simulink model "uz_sine_generator_16bit"  (R2023a)
settings: Solver=FixedStepDiscrete  StartTime=0.0  StopTime=50000/100e6  RelTol=1e-3
libraries: hdlsllib x17, embmathops x8, simulink x1
settings Model: DataTypeOverride=Off  Creator=ts  LastModifiedBy=ts
settings SolverCC: AlgebraicLoopSolver=TrustRegion
settings DataIOCC: LimitDataPoints=on  SaveOutput=off  SaveTime=off
settings OptimizationCC: BlockReduction=off  ConditionallyExecuteInputs=off  DefaultParameterBehavior=Inlined  LifeSpan=inf
settings DebuggingCC: AlgebraicLoopMsg=error  SingleTaskRateTransMsg=error  UnconnectedInputMsg=warning  UnconnectedOutputMsg=warning  UnconnectedLineMsg=warning  AllowSymbolicDim=off  StrictBusMsg=ErrorOnBusTreatedAsVector  SFUnexpectedBacktrackingDiag=warning  SFNoUnconditionalDefaultTransitionDiag=warning  SFExecutionAtInitializationDiag=none  ArithmeticOperatorsInVariantConditions=warning
settings HardwareCC: ProdBitPerPointer=32  ProdBitPerSizeT=32  ProdBitPerPtrDiffT=32  ProdLargestAtomicFloat=None  ProdIntDivRoundTo=Undefined  ProdEndianess=Unspecified  ProdWordSize=32  ProdHWDeviceType=ASIC/FPGA->ASIC/FPGA  ProdEqTarget=off
settings ModelReferenceCC: EnableRefExpFcnMdlSchedulingChecks=on
settings SFSimCC: SimUseLocalCustomCode=off  CustomCodeUndefinedFunction=UseInterfaceOnly
settings RTWCC: RTWUseLocalCustomCode=off
settings CodeAppCC: StateflowObjectComments=on
settings GRTTargetCC: TargetLangStandard=C89/C90 (ANSI)
settings ConfigComp: CovScope=ReferencedModels  CovMetricSettings=dw  CovSaveCumulativeToWorkspaceVar=on  CovSaveSingleToWorkspaceVar=on  CovExternalEMLEnable=off  CovSFcnEnable=off

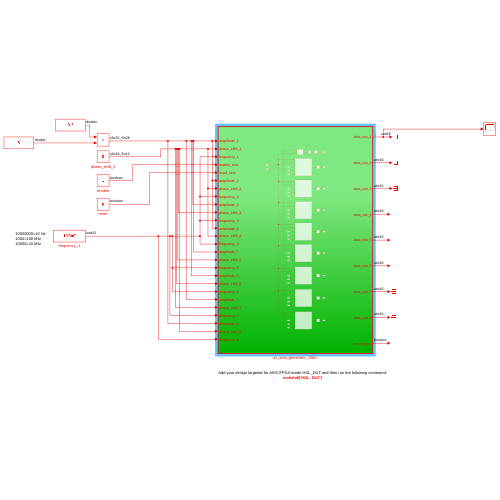
[thumbnail: Simulink's stored preview of the top-level diagram]
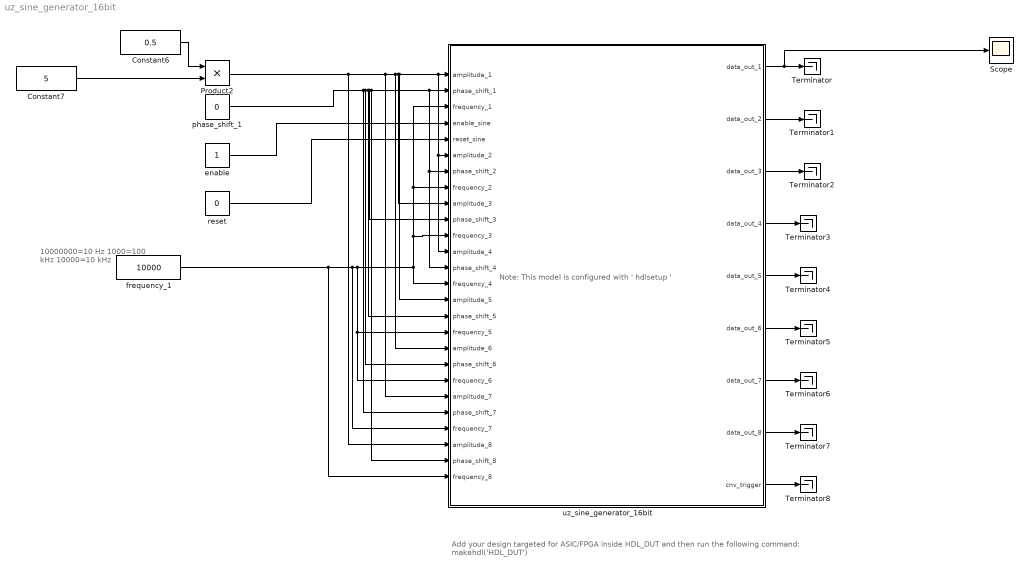
== system uz_sine_generator_16bit ==
  note: Note: This model is configured with ' hdlsetup '
  note: Add your design targeted for ASIC/FPGA inside HDL_DUT and then run the following command:
      | makehdl('HDL_DUT')
  note: 10000000=10 Hz
      | 1000=100 kHz
      | 10000=10 kHz
  Constant6 : Constant  Value=0.5  SampleTime=-1
  Constant7 : Constant  Value=5  SampleTime=-1
  Product2 : Product  OutDataTypeStr=fixdt(1,32,28)
  Scope : Scope
  Terminator{,1..8} (9 alike) : Terminator
  enable : Constant  OutDataTypeStr=boolean  SampleTime=-1
  frequency_1 : Constant  Value=10000  OutDataTypeStr=uint32  SampleTime=1/100e6
  phase_shift_1 : Constant  Value=0  OutDataTypeStr=fixdt(1,16,12)  SampleTime=-1
  reset : Constant  Value=0  OutDataTypeStr=boolean  SampleTime=-1
  "uz_sine_generator_16bit " : Subsystem  TreatAsAtomicUnit=on
  wires:
  Constant6/1 -> Product2/1
  Constant7/1 -> Product2/2
  Product2/1 -> "uz_sine_generator_16bit "/24(amplitude_8), "uz_sine_generator_16bit "/21(amplitude_7), "uz_sine_generator_16bit "/18(amplitude_6), "uz_sine_generator_16bit "/9(amplitude_3), "uz_sine_generator_16bit "/15(amplitude_5), "uz_sine_generator_16bit "/12(amplitude_4), "uz_sine_generator_16bit "/6(amplitude_2), "uz_sine_generator_16bit "/1(amplitude_1)
  phase_shift_1/1 -> "uz_sine_generator_16bit "/25(phase_shift_8), "uz_sine_generator_16bit "/13(phase_shift_4), "uz_sine_generator_16bit "/7(phase_shift_2), "uz_sine_generator_16bit "/2(phase_shift_1), "uz_sine_generator_16bit "/10(phase_shift_3), "uz_sine_generator_16bit "/16(phase_shift_5), "uz_sine_generator_16bit "/19(phase_shift_6), "uz_sine_generator_16bit "/22(phase_shift_7)
  "uz_sine_generator_16bit "/1(data_out_1) -> Scope/1, Terminator/1
  "uz_sine_generator_16bit "/2(data_out_2) -> Terminator1/1
  "uz_sine_generator_16bit "/3(data_out_3) -> Terminator2/1
  "uz_sine_generator_16bit "/4(data_out_4) -> Terminator3/1
  "uz_sine_generator_16bit "/5(data_out_5) -> Terminator4/1
  "uz_sine_generator_16bit "/6(data_out_6) -> Terminator5/1
  "uz_sine_generator_16bit "/7(data_out_7) -> Terminator6/1
  "uz_sine_generator_16bit "/8(data_out_8) -> Terminator7/1
  "uz_sine_generator_16bit "/9(cnv_trigger) -> Terminator8/1
  enable/1 -> "uz_sine_generator_16bit "/4(enable_sine)
  reset/1 -> "uz_sine_generator_16bit "/5(reset_sine)
  frequency_1/1 -> "uz_sine_generator_16bit "/26(frequency_8), "uz_sine_generator_16bit "/23(frequency_7), "uz_sine_generator_16bit "/20(frequency_6), "uz_sine_generator_16bit "/17(frequency_5), "uz_sine_generator_16bit "/14(frequency_4), "uz_sine_generator_16bit "/11(frequency_3), "uz_sine_generator_16bit "/3(frequency_1), "uz_sine_generator_16bit "/8(frequency_2)

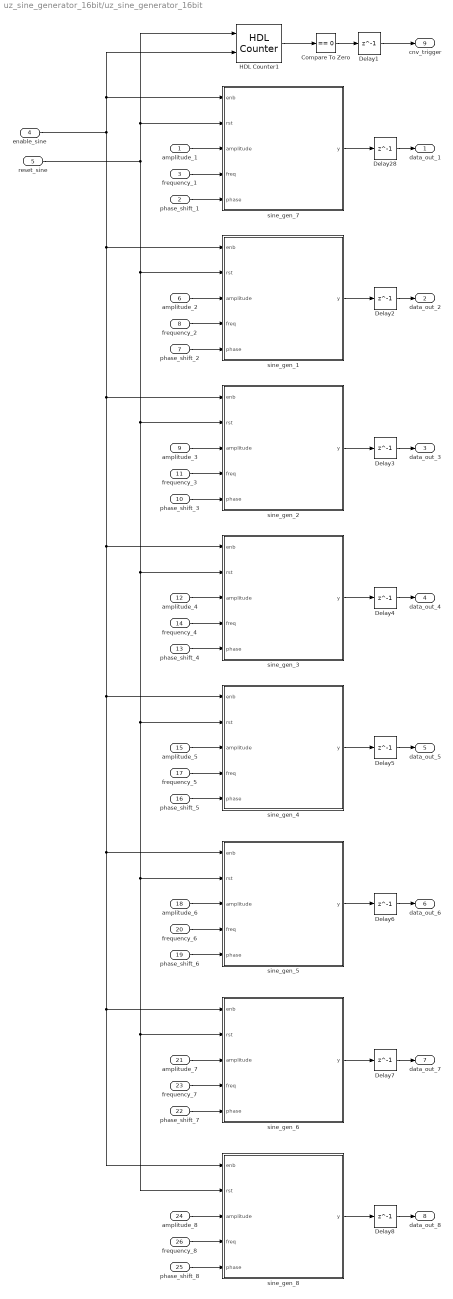
== system uz_sine_generator_16bit/uz_sine_generator_16bit  ==
  amplitude_1 : Inport
  phase_shift_1 : Inport  Port=2
  frequency_1 : Inport  Port=3
  enable_sine : Inport  Port=4
  reset_sine : Inport  Port=5
  amplitude_2 : Inport  Port=6
  phase_shift_2 : Inport  Port=7
  frequency_2 : Inport  Port=8
  amplitude_3 : Inport  Port=9
  phase_shift_3 : Inport  Port=10
  frequency_3 : Inport  Port=11
  amplitude_4 : Inport  Port=12
  phase_shift_4 : Inport  Port=13
  frequency_4 : Inport  Port=14
  amplitude_5 : Inport  Port=15
  phase_shift_5 : Inport  Port=16
  frequency_5 : Inport  Port=17
  amplitude_6 : Inport  Port=18
  phase_shift_6 : Inport  Port=19
  frequency_6 : Inport  Port=20
  amplitude_7 : Inport  Port=21
  phase_shift_7 : Inport  Port=22
  frequency_7 : Inport  Port=23
  amplitude_8 : Inport  Port=24
  phase_shift_8 : Inport  Port=25
  frequency_8 : Inport  Port=26
  Compare To Zero : simulink/Logic and Bit Operations/Compare To Zero  relop===  OutDataTypeStr=boolean
  Delay{1..8,28} (9 alike) : Delay  DelayLength=1
  HDL Counter1 : hdlsllib/Sources/HDL Counter  CountType=Free running  CountInit=0  CountStep=100  CountMax=25  CountFromType=Initial value  CountFrom=0  CountResetPort=on  CountLoadPort=off  CountEnbPort=on  CountDirPort=off  CountHitOutputPort=off  CountDataType=Unsigned  CountWordLen=8  CountFracLen=0  CountSampTime=1
  sine_gen_1 : Subsystem
  sine_gen_2 : Subsystem
  sine_gen_3 : Subsystem
  sine_gen_4 : Subsystem
  sine_gen_5 : Subsystem
  sine_gen_6 : Subsystem
  sine_gen_7 : Subsystem
  sine_gen_8 : Subsystem
  data_out_1 : Outport  VectorParamsAs1DForOutWhenUnconnected=off
  data_out_2 : Outport  Port=2  VectorParamsAs1DForOutWhenUnconnected=off
  data_out_3 : Outport  Port=3  VectorParamsAs1DForOutWhenUnconnected=off
  data_out_4 : Outport  Port=4  VectorParamsAs1DForOutWhenUnconnected=off
  data_out_5 : Outport  Port=5  VectorParamsAs1DForOutWhenUnconnected=off
  data_out_6 : Outport  Port=6  VectorParamsAs1DForOutWhenUnconnected=off
  data_out_7 : Outport  Port=7  VectorParamsAs1DForOutWhenUnconnected=off
  data_out_8 : Outport  Port=8  VectorParamsAs1DForOutWhenUnconnected=off
  cnv_trigger : Outport  Port=9  VectorParamsAs1DForOutWhenUnconnected=off
  wires:
  Delay28/1 -> data_out_1/1
  HDL Counter1/1 -> Compare To Zero/1
  Compare To Zero/1 -> Delay1/1
  sine_gen_7/1(y) -> Delay28/1
  amplitude_1/1 -> sine_gen_7/3(amplitude)
  Delay1/1 -> cnv_trigger/1
  amplitude_2/1 -> sine_gen_1/3(amplitude)
  sine_gen_1/1(y) -> Delay2/1
  Delay2/1 -> data_out_2/1
  amplitude_3/1 -> sine_gen_2/3(amplitude)
  sine_gen_2/1(y) -> Delay3/1
  Delay3/1 -> data_out_3/1
  amplitude_4/1 -> sine_gen_3/3(amplitude)
  sine_gen_3/1(y) -> Delay4/1
  Delay4/1 -> data_out_4/1
  amplitude_5/1 -> sine_gen_4/3(amplitude)
  sine_gen_4/1(y) -> Delay5/1
  Delay5/1 -> data_out_5/1
  amplitude_6/1 -> sine_gen_5/3(amplitude)
  sine_gen_5/1(y) -> Delay6/1
  Delay6/1 -> data_out_6/1
  amplitude_7/1 -> sine_gen_6/3(amplitude)
  sine_gen_6/1(y) -> Delay7/1
  Delay7/1 -> data_out_7/1
  amplitude_8/1 -> sine_gen_8/3(amplitude)
  sine_gen_8/1(y) -> Delay8/1
  enable_sine/1 -> sine_gen_7/1(enb), HDL Counter1/2, sine_gen_1/1(enb), sine_gen_2/1(enb), sine_gen_3/1(enb), sine_gen_4/1(enb), sine_gen_5/1(enb), sine_gen_8/1(enb), sine_gen_6/1(enb)
  reset_sine/1 -> sine_gen_1/2(rst), sine_gen_2/2(rst), sine_gen_3/2(rst), sine_gen_4/2(rst), sine_gen_5/2(rst), sine_gen_8/2(rst), sine_gen_6/2(rst), sine_gen_7/2(rst), HDL Counter1/1
  Delay8/1 -> data_out_8/1
  frequency_1/1 -> sine_gen_7/4(freq)
  phase_shift_1/1 -> sine_gen_7/5(phase)
  frequency_2/1 -> sine_gen_1/4(freq)
  phase_shift_2/1 -> sine_gen_1/5(phase)
  frequency_3/1 -> sine_gen_2/4(freq)
  phase_shift_3/1 -> sine_gen_2/5(phase)
  frequency_4/1 -> sine_gen_3/4(freq)
  phase_shift_4/1 -> sine_gen_3/5(phase)
  frequency_5/1 -> sine_gen_4/4(freq)
  phase_shift_5/1 -> sine_gen_4/5(phase)
  frequency_6/1 -> sine_gen_5/4(freq)
  phase_shift_6/1 -> sine_gen_5/5(phase)
  frequency_7/1 -> sine_gen_6/4(freq)
  phase_shift_7/1 -> sine_gen_6/5(phase)
  frequency_8/1 -> sine_gen_8/4(freq)
  phase_shift_8/1 -> sine_gen_8/5(phase)

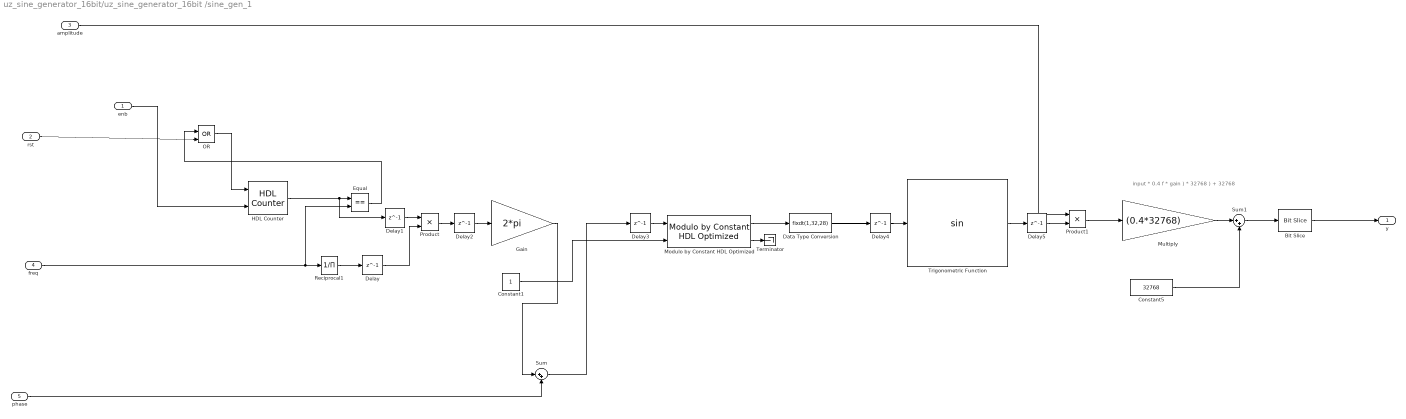
== system uz_sine_generator_16bit/uz_sine_generator_16bit /sine_gen_1 ==
  note: input * 0.4 f * gain ) * 32768 ) + 32768
  enb : Inport
  rst : Inport  Port=2
  amplitude : Inport  Port=3
  freq : Inport  Port=4
  phase : Inport  Port=5
  Bit Slice : hdlsllib/Logic and Bit Operations/Bit Slice  lidx=15  ridx=0
  Constant1 : Constant  OutDataTypeStr=boolean  SampleTime=-1
  Constant5 : Constant  Value=32768  OutDataTypeStr=int32  SampleTime=-1
  Data Type Conversion : DataTypeConversion  OutDataTypeStr=fixdt(1,32,28)  SaturateOnIntegerOverflow=off  RndMeth=Floor
  Delay{,1..5} (6 alike) : Delay  DelayLength=1
  Equal : RelationalOperator  Operator===  OutDataTypeStr=boolean  RndMeth=Simplest  InputSameDT=off
  Gain : Gain  Gain=2*pi  OutDataTypeStr=fixdt(1,32,28)
  HDL Counter : hdlsllib/Sources/HDL Counter  CountType=Free running  CountInit=0  CountStep=1  CountMax=25  CountFromType=Initial value  CountFrom=0  CountResetPort=on  CountLoadPort=off  CountEnbPort=on  CountDirPort=off  CountHitOutputPort=off  CountDataType=Unsigned  CountWordLen=32  CountFracLen=0  CountSampTime=1
  Modulo by Constant HDL Optimized : embmathops/Modulo by Constant HDL Optimized  Denominator=2*pi  SimulateUsing=Code generation
      settings: LibrarySourceBlock=|
      | embeddedMatrixLib/Math Operations/Modulo by Constant
      | HDL Optimized
  Multiply : Gain  Gain=(0.4*32768)  OutDataTypeStr=int32
  OR : Logic  Operator=OR  IconShape=distinctive  AllPortsSameDT=off  OutDataTypeStr=boolean
  Product : Product  OutDataTypeStr=fixdt(0,32,29)
  Product1 : Product  OutDataTypeStr=Inherit: Same as first input
  Reciprocal1 : Product  Inputs=/  RndMeth=Zero  SaturateOnIntegerOverflow=on
  Sum : Sum  Inputs=|++
  Sum1 : Sum  Inputs=|++  OutDataTypeStr=int32
  Terminator : Terminator
  Trigonometric Function : Trigonometry  ApproximationMethod=CORDIC
  y : Outport
  wires:
  Constant1/1 -> Modulo by Constant HDL Optimized/2
  Product1/1 -> Multiply/1
  Constant5/1 -> Sum1/2
  Gain/1 -> Sum/1
  Sum/1 -> Delay3/1
  Modulo by Constant HDL Optimized/1 -> Data Type Conversion/1
  freq/1 -> Reciprocal1/1, Equal/2
  Reciprocal1/1 -> Delay/1
  amplitude/1 -> Product1/1
  Sum1/1 -> Bit Slice/1
  phase/1 -> Sum/2
  Product/1 -> Delay2/1
  Equal/1 -> OR/1
  Trigonometric Function/1 -> Delay5/1
  enb/1 -> HDL Counter/2
  Multiply/1 -> Sum1/1
  Bit Slice/1 -> y/1
  Modulo by Constant HDL Optimized/2 -> Terminator/1
  OR/1 -> HDL Counter/1
  rst/1 -> OR/2
  HDL Counter/1 -> Delay1/1, Equal/1
  Data Type Conversion/1 -> Delay4/1
  Delay/1 -> Product/2
  Delay1/1 -> Product/1
  Delay2/1 -> Gain/1
  Delay3/1 -> Modulo by Constant HDL Optimized/1
  Delay4/1 -> Trigonometric Function/1
  Delay5/1 -> Product1/2

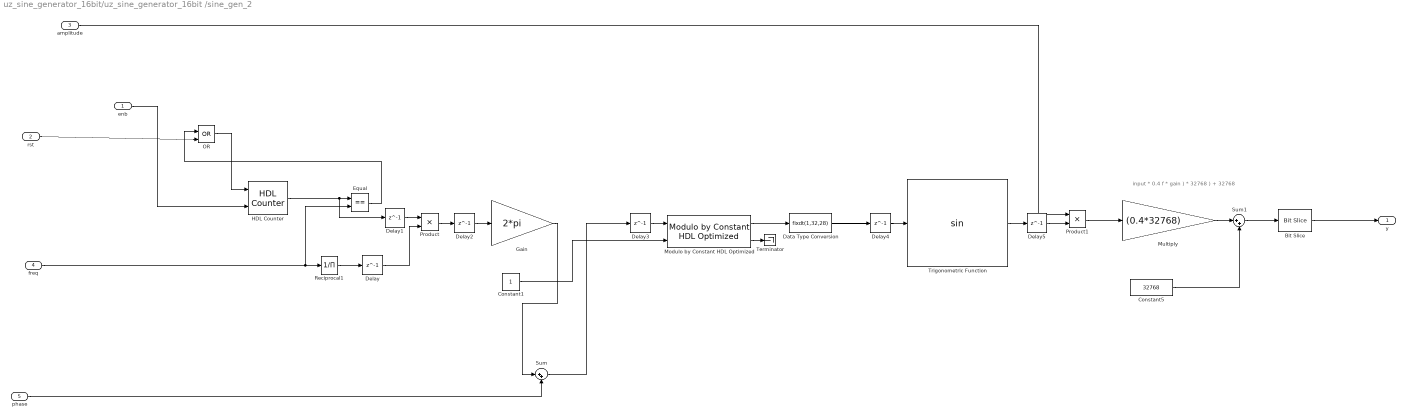
== system uz_sine_generator_16bit/uz_sine_generator_16bit /sine_gen_2 ==
  note: input * 0.4 f * gain ) * 32768 ) + 32768
  enb : Inport
  rst : Inport  Port=2
  amplitude : Inport  Port=3
  freq : Inport  Port=4
  phase : Inport  Port=5
  Bit Slice : hdlsllib/Logic and Bit Operations/Bit Slice  lidx=15  ridx=0
  Constant1 : Constant  OutDataTypeStr=boolean  SampleTime=-1
  Constant5 : Constant  Value=32768  OutDataTypeStr=int32  SampleTime=-1
  Data Type Conversion : DataTypeConversion  OutDataTypeStr=fixdt(1,32,28)  SaturateOnIntegerOverflow=off  RndMeth=Floor
  Delay{,1..5} (6 alike) : Delay  DelayLength=1
  Equal : RelationalOperator  Operator===  OutDataTypeStr=boolean  RndMeth=Simplest  InputSameDT=off
  Gain : Gain  Gain=2*pi  OutDataTypeStr=fixdt(1,32,28)
  HDL Counter : hdlsllib/Sources/HDL Counter  CountType=Free running  CountInit=0  CountStep=1  CountMax=25  CountFromType=Initial value  CountFrom=0  CountResetPort=on  CountLoadPort=off  CountEnbPort=on  CountDirPort=off  CountHitOutputPort=off  CountDataType=Unsigned  CountWordLen=32  CountFracLen=0  CountSampTime=1
  Modulo by Constant HDL Optimized : embmathops/Modulo by Constant HDL Optimized  Denominator=2*pi  SimulateUsing=Code generation
      settings: LibrarySourceBlock=|
      | embeddedMatrixLib/Math Operations/Modulo by Constant
      | HDL Optimized
  Multiply : Gain  Gain=(0.4*32768)  OutDataTypeStr=int32
  OR : Logic  Operator=OR  IconShape=distinctive  AllPortsSameDT=off  OutDataTypeStr=boolean
  Product : Product  OutDataTypeStr=fixdt(0,32,29)
  Product1 : Product  OutDataTypeStr=Inherit: Same as first input
  Reciprocal1 : Product  Inputs=/  RndMeth=Zero  SaturateOnIntegerOverflow=on
  Sum : Sum  Inputs=|++
  Sum1 : Sum  Inputs=|++  OutDataTypeStr=int32
  Terminator : Terminator
  Trigonometric Function : Trigonometry  ApproximationMethod=CORDIC
  y : Outport
  wires:
  Constant1/1 -> Modulo by Constant HDL Optimized/2
  Product1/1 -> Multiply/1
  Constant5/1 -> Sum1/2
  Gain/1 -> Sum/1
  Sum/1 -> Delay3/1
  Modulo by Constant HDL Optimized/1 -> Data Type Conversion/1
  freq/1 -> Reciprocal1/1, Equal/2
  Reciprocal1/1 -> Delay/1
  amplitude/1 -> Product1/1
  Sum1/1 -> Bit Slice/1
  phase/1 -> Sum/2
  Product/1 -> Delay2/1
  Equal/1 -> OR/1
  Trigonometric Function/1 -> Delay5/1
  enb/1 -> HDL Counter/2
  Multiply/1 -> Sum1/1
  Bit Slice/1 -> y/1
  Modulo by Constant HDL Optimized/2 -> Terminator/1
  OR/1 -> HDL Counter/1
  rst/1 -> OR/2
  HDL Counter/1 -> Delay1/1, Equal/1
  Data Type Conversion/1 -> Delay4/1
  Delay/1 -> Product/2
  Delay1/1 -> Product/1
  Delay2/1 -> Gain/1
  Delay3/1 -> Modulo by Constant HDL Optimized/1
  Delay4/1 -> Trigonometric Function/1
  Delay5/1 -> Product1/2

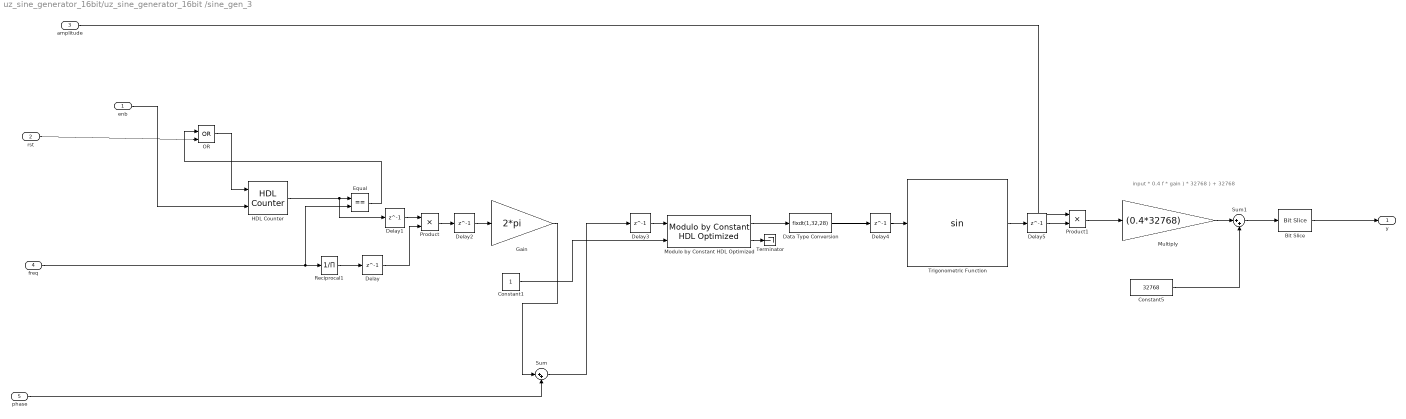
== system uz_sine_generator_16bit/uz_sine_generator_16bit /sine_gen_3 ==
  note: input * 0.4 f * gain ) * 32768 ) + 32768
  enb : Inport
  rst : Inport  Port=2
  amplitude : Inport  Port=3
  freq : Inport  Port=4
  phase : Inport  Port=5
  Bit Slice : hdlsllib/Logic and Bit Operations/Bit Slice  lidx=15  ridx=0
  Constant1 : Constant  OutDataTypeStr=boolean  SampleTime=-1
  Constant5 : Constant  Value=32768  OutDataTypeStr=int32  SampleTime=-1
  Data Type Conversion : DataTypeConversion  OutDataTypeStr=fixdt(1,32,28)  SaturateOnIntegerOverflow=off  RndMeth=Floor
  Delay{,1..5} (6 alike) : Delay  DelayLength=1
  Equal : RelationalOperator  Operator===  OutDataTypeStr=boolean  RndMeth=Simplest  InputSameDT=off
  Gain : Gain  Gain=2*pi  OutDataTypeStr=fixdt(1,32,28)
  HDL Counter : hdlsllib/Sources/HDL Counter  CountType=Free running  CountInit=0  CountStep=1  CountMax=25  CountFromType=Initial value  CountFrom=0  CountResetPort=on  CountLoadPort=off  CountEnbPort=on  CountDirPort=off  CountHitOutputPort=off  CountDataType=Unsigned  CountWordLen=32  CountFracLen=0  CountSampTime=1
  Modulo by Constant HDL Optimized : embmathops/Modulo by Constant HDL Optimized  Denominator=2*pi  SimulateUsing=Code generation
      settings: LibrarySourceBlock=|
      | embeddedMatrixLib/Math Operations/Modulo by Constant
      | HDL Optimized
  Multiply : Gain  Gain=(0.4*32768)  OutDataTypeStr=int32
  OR : Logic  Operator=OR  IconShape=distinctive  AllPortsSameDT=off  OutDataTypeStr=boolean
  Product : Product  OutDataTypeStr=fixdt(0,32,29)
  Product1 : Product  OutDataTypeStr=Inherit: Same as first input
  Reciprocal1 : Product  Inputs=/  RndMeth=Zero  SaturateOnIntegerOverflow=on
  Sum : Sum  Inputs=|++
  Sum1 : Sum  Inputs=|++  OutDataTypeStr=int32
  Terminator : Terminator
  Trigonometric Function : Trigonometry  ApproximationMethod=CORDIC
  y : Outport
  wires:
  Constant1/1 -> Modulo by Constant HDL Optimized/2
  Product1/1 -> Multiply/1
  Constant5/1 -> Sum1/2
  Gain/1 -> Sum/1
  Sum/1 -> Delay3/1
  Modulo by Constant HDL Optimized/1 -> Data Type Conversion/1
  freq/1 -> Reciprocal1/1, Equal/2
  Reciprocal1/1 -> Delay/1
  amplitude/1 -> Product1/1
  Sum1/1 -> Bit Slice/1
  phase/1 -> Sum/2
  Product/1 -> Delay2/1
  Equal/1 -> OR/1
  Trigonometric Function/1 -> Delay5/1
  enb/1 -> HDL Counter/2
  Multiply/1 -> Sum1/1
  Bit Slice/1 -> y/1
  Modulo by Constant HDL Optimized/2 -> Terminator/1
  OR/1 -> HDL Counter/1
  rst/1 -> OR/2
  HDL Counter/1 -> Delay1/1, Equal/1
  Data Type Conversion/1 -> Delay4/1
  Delay/1 -> Product/2
  Delay1/1 -> Product/1
  Delay2/1 -> Gain/1
  Delay3/1 -> Modulo by Constant HDL Optimized/1
  Delay4/1 -> Trigonometric Function/1
  Delay5/1 -> Product1/2

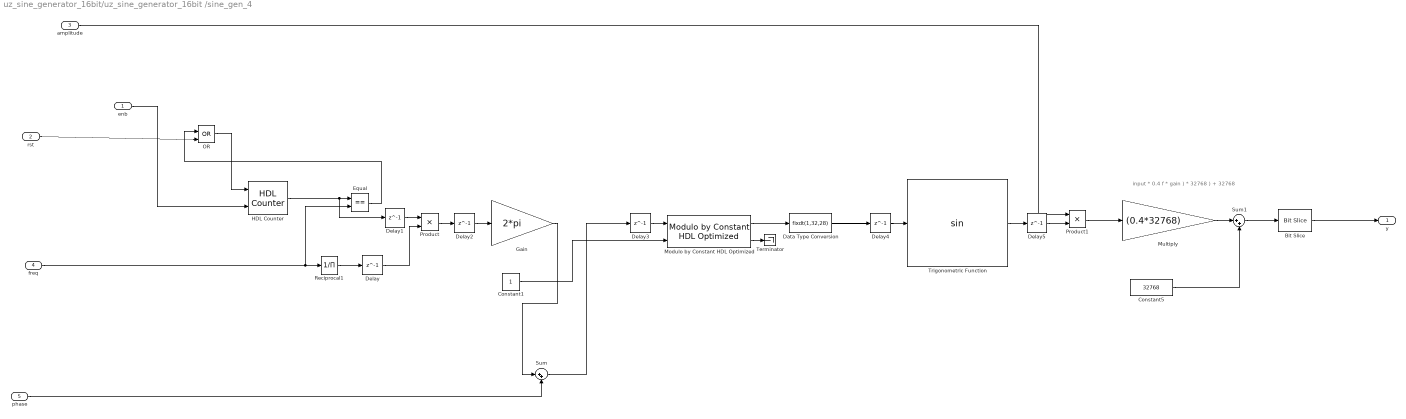
== system uz_sine_generator_16bit/uz_sine_generator_16bit /sine_gen_4 ==
  note: input * 0.4 f * gain ) * 32768 ) + 32768
  enb : Inport
  rst : Inport  Port=2
  amplitude : Inport  Port=3
  freq : Inport  Port=4
  phase : Inport  Port=5
  Bit Slice : hdlsllib/Logic and Bit Operations/Bit Slice  lidx=15  ridx=0
  Constant1 : Constant  OutDataTypeStr=boolean  SampleTime=-1
  Constant5 : Constant  Value=32768  OutDataTypeStr=int32  SampleTime=-1
  Data Type Conversion : DataTypeConversion  OutDataTypeStr=fixdt(1,32,28)  SaturateOnIntegerOverflow=off  RndMeth=Floor
  Delay{,1..5} (6 alike) : Delay  DelayLength=1
  Equal : RelationalOperator  Operator===  OutDataTypeStr=boolean  RndMeth=Simplest  InputSameDT=off
  Gain : Gain  Gain=2*pi  OutDataTypeStr=fixdt(1,32,28)
  HDL Counter : hdlsllib/Sources/HDL Counter  CountType=Free running  CountInit=0  CountStep=1  CountMax=25  CountFromType=Initial value  CountFrom=0  CountResetPort=on  CountLoadPort=off  CountEnbPort=on  CountDirPort=off  CountHitOutputPort=off  CountDataType=Unsigned  CountWordLen=32  CountFracLen=0  CountSampTime=1
  Modulo by Constant HDL Optimized : embmathops/Modulo by Constant HDL Optimized  Denominator=2*pi  SimulateUsing=Code generation
      settings: LibrarySourceBlock=|
      | embeddedMatrixLib/Math Operations/Modulo by Constant
      | HDL Optimized
  Multiply : Gain  Gain=(0.4*32768)  OutDataTypeStr=int32
  OR : Logic  Operator=OR  IconShape=distinctive  AllPortsSameDT=off  OutDataTypeStr=boolean
  Product : Product  OutDataTypeStr=fixdt(0,32,29)
  Product1 : Product  OutDataTypeStr=Inherit: Same as first input
  Reciprocal1 : Product  Inputs=/  RndMeth=Zero  SaturateOnIntegerOverflow=on
  Sum : Sum  Inputs=|++
  Sum1 : Sum  Inputs=|++  OutDataTypeStr=int32
  Terminator : Terminator
  Trigonometric Function : Trigonometry  ApproximationMethod=CORDIC
  y : Outport
  wires:
  Constant1/1 -> Modulo by Constant HDL Optimized/2
  Product1/1 -> Multiply/1
  Constant5/1 -> Sum1/2
  Gain/1 -> Sum/1
  Sum/1 -> Delay3/1
  Modulo by Constant HDL Optimized/1 -> Data Type Conversion/1
  freq/1 -> Reciprocal1/1, Equal/2
  Reciprocal1/1 -> Delay/1
  amplitude/1 -> Product1/1
  Sum1/1 -> Bit Slice/1
  phase/1 -> Sum/2
  Product/1 -> Delay2/1
  Equal/1 -> OR/1
  Trigonometric Function/1 -> Delay5/1
  enb/1 -> HDL Counter/2
  Multiply/1 -> Sum1/1
  Bit Slice/1 -> y/1
  Modulo by Constant HDL Optimized/2 -> Terminator/1
  OR/1 -> HDL Counter/1
  rst/1 -> OR/2
  HDL Counter/1 -> Delay1/1, Equal/1
  Data Type Conversion/1 -> Delay4/1
  Delay/1 -> Product/2
  Delay1/1 -> Product/1
  Delay2/1 -> Gain/1
  Delay3/1 -> Modulo by Constant HDL Optimized/1
  Delay4/1 -> Trigonometric Function/1
  Delay5/1 -> Product1/2

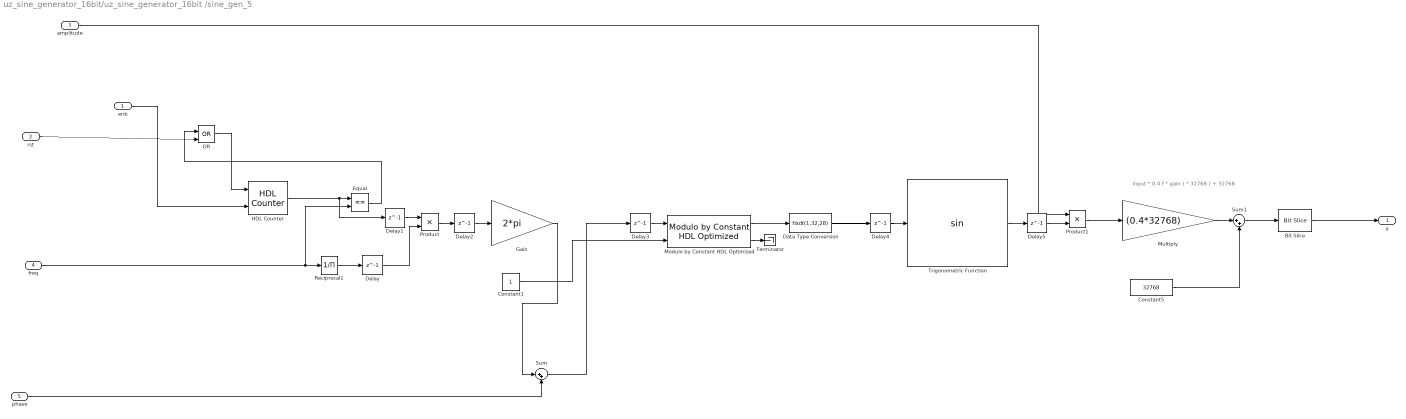
== system uz_sine_generator_16bit/uz_sine_generator_16bit /sine_gen_5 ==
  note: input * 0.4 f * gain ) * 32768 ) + 32768
  enb : Inport
  rst : Inport  Port=2
  amplitude : Inport  Port=3
  freq : Inport  Port=4
  phase : Inport  Port=5
  Bit Slice : hdlsllib/Logic and Bit Operations/Bit Slice  lidx=15  ridx=0
  Constant1 : Constant  OutDataTypeStr=boolean  SampleTime=-1
  Constant5 : Constant  Value=32768  OutDataTypeStr=int32  SampleTime=-1
  Data Type Conversion : DataTypeConversion  OutDataTypeStr=fixdt(1,32,28)  SaturateOnIntegerOverflow=off  RndMeth=Floor
  Delay{,1..5} (6 alike) : Delay  DelayLength=1
  Equal : RelationalOperator  Operator===  OutDataTypeStr=boolean  RndMeth=Simplest  InputSameDT=off
  Gain : Gain  Gain=2*pi  OutDataTypeStr=fixdt(1,32,28)
  HDL Counter : hdlsllib/Sources/HDL Counter  CountType=Free running  CountInit=0  CountStep=1  CountMax=25  CountFromType=Initial value  CountFrom=0  CountResetPort=on  CountLoadPort=off  CountEnbPort=on  CountDirPort=off  CountHitOutputPort=off  CountDataType=Unsigned  CountWordLen=32  CountFracLen=0  CountSampTime=1
  Modulo by Constant HDL Optimized : embmathops/Modulo by Constant HDL Optimized  Denominator=2*pi  SimulateUsing=Code generation
      settings: LibrarySourceBlock=|
      | embeddedMatrixLib/Math Operations/Modulo by Constant
      | HDL Optimized
  Multiply : Gain  Gain=(0.4*32768)  OutDataTypeStr=int32
  OR : Logic  Operator=OR  IconShape=distinctive  AllPortsSameDT=off  OutDataTypeStr=boolean
  Product : Product  OutDataTypeStr=fixdt(0,32,29)
  Product1 : Product  OutDataTypeStr=Inherit: Same as first input
  Reciprocal1 : Product  Inputs=/  RndMeth=Zero  SaturateOnIntegerOverflow=on
  Sum : Sum  Inputs=|++
  Sum1 : Sum  Inputs=|++  OutDataTypeStr=int32
  Terminator : Terminator
  Trigonometric Function : Trigonometry  ApproximationMethod=CORDIC
  y : Outport
  wires:
  Constant1/1 -> Modulo by Constant HDL Optimized/2
  Product1/1 -> Multiply/1
  Constant5/1 -> Sum1/2
  Gain/1 -> Sum/1
  Sum/1 -> Delay3/1
  Modulo by Constant HDL Optimized/1 -> Data Type Conversion/1
  freq/1 -> Reciprocal1/1, Equal/2
  Reciprocal1/1 -> Delay/1
  amplitude/1 -> Product1/1
  Sum1/1 -> Bit Slice/1
  phase/1 -> Sum/2
  Product/1 -> Delay2/1
  Equal/1 -> OR/1
  Trigonometric Function/1 -> Delay5/1
  enb/1 -> HDL Counter/2
  Multiply/1 -> Sum1/1
  Bit Slice/1 -> y/1
  Modulo by Constant HDL Optimized/2 -> Terminator/1
  OR/1 -> HDL Counter/1
  rst/1 -> OR/2
  HDL Counter/1 -> Delay1/1, Equal/1
  Data Type Conversion/1 -> Delay4/1
  Delay/1 -> Product/2
  Delay1/1 -> Product/1
  Delay2/1 -> Gain/1
  Delay3/1 -> Modulo by Constant HDL Optimized/1
  Delay4/1 -> Trigonometric Function/1
  Delay5/1 -> Product1/2

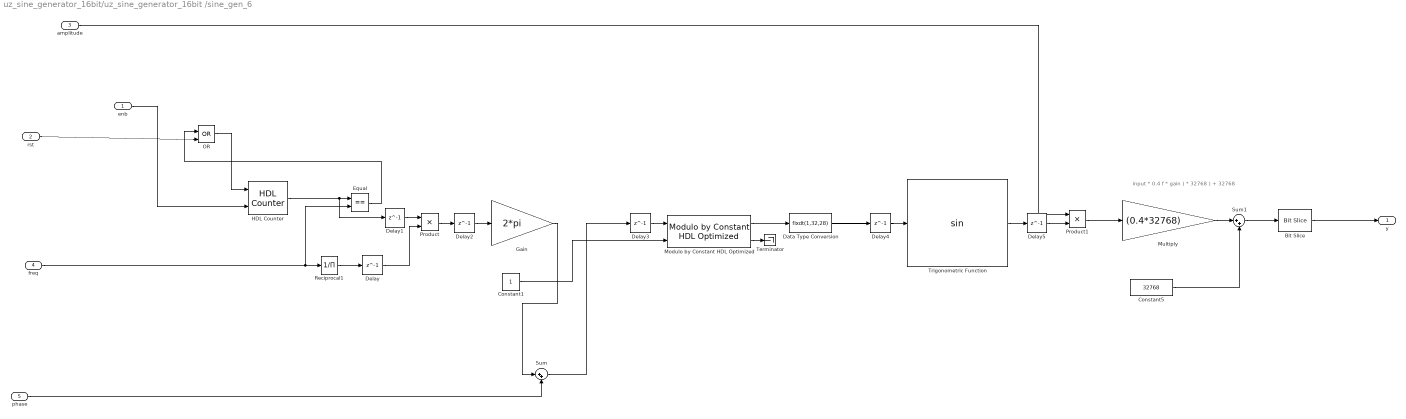
== system uz_sine_generator_16bit/uz_sine_generator_16bit /sine_gen_6 ==
  note: input * 0.4 f * gain ) * 32768 ) + 32768
  enb : Inport
  rst : Inport  Port=2
  amplitude : Inport  Port=3
  freq : Inport  Port=4
  phase : Inport  Port=5
  Bit Slice : hdlsllib/Logic and Bit Operations/Bit Slice  lidx=15  ridx=0
  Constant1 : Constant  OutDataTypeStr=boolean  SampleTime=-1
  Constant5 : Constant  Value=32768  OutDataTypeStr=int32  SampleTime=-1
  Data Type Conversion : DataTypeConversion  OutDataTypeStr=fixdt(1,32,28)  SaturateOnIntegerOverflow=off  RndMeth=Floor
  Delay{,1..5} (6 alike) : Delay  DelayLength=1
  Equal : RelationalOperator  Operator===  OutDataTypeStr=boolean  RndMeth=Simplest  InputSameDT=off
  Gain : Gain  Gain=2*pi  OutDataTypeStr=fixdt(1,32,28)
  HDL Counter : hdlsllib/Sources/HDL Counter  CountType=Free running  CountInit=0  CountStep=1  CountMax=25  CountFromType=Initial value  CountFrom=0  CountResetPort=on  CountLoadPort=off  CountEnbPort=on  CountDirPort=off  CountHitOutputPort=off  CountDataType=Unsigned  CountWordLen=32  CountFracLen=0  CountSampTime=1
  Modulo by Constant HDL Optimized : embmathops/Modulo by Constant HDL Optimized  Denominator=2*pi  SimulateUsing=Code generation
      settings: LibrarySourceBlock=|
      | embeddedMatrixLib/Math Operations/Modulo by Constant
      | HDL Optimized
  Multiply : Gain  Gain=(0.4*32768)  OutDataTypeStr=int32
  OR : Logic  Operator=OR  IconShape=distinctive  AllPortsSameDT=off  OutDataTypeStr=boolean
  Product : Product  OutDataTypeStr=fixdt(0,32,29)
  Product1 : Product  OutDataTypeStr=Inherit: Same as first input
  Reciprocal1 : Product  Inputs=/  RndMeth=Zero  SaturateOnIntegerOverflow=on
  Sum : Sum  Inputs=|++
  Sum1 : Sum  Inputs=|++  OutDataTypeStr=int32
  Terminator : Terminator
  Trigonometric Function : Trigonometry  ApproximationMethod=CORDIC
  y : Outport
  wires:
  Constant1/1 -> Modulo by Constant HDL Optimized/2
  Product1/1 -> Multiply/1
  Constant5/1 -> Sum1/2
  Gain/1 -> Sum/1
  Sum/1 -> Delay3/1
  Modulo by Constant HDL Optimized/1 -> Data Type Conversion/1
  freq/1 -> Reciprocal1/1, Equal/2
  Reciprocal1/1 -> Delay/1
  amplitude/1 -> Product1/1
  Sum1/1 -> Bit Slice/1
  phase/1 -> Sum/2
  Product/1 -> Delay2/1
  Equal/1 -> OR/1
  Trigonometric Function/1 -> Delay5/1
  enb/1 -> HDL Counter/2
  Multiply/1 -> Sum1/1
  Bit Slice/1 -> y/1
  Modulo by Constant HDL Optimized/2 -> Terminator/1
  OR/1 -> HDL Counter/1
  rst/1 -> OR/2
  HDL Counter/1 -> Delay1/1, Equal/1
  Data Type Conversion/1 -> Delay4/1
  Delay/1 -> Product/2
  Delay1/1 -> Product/1
  Delay2/1 -> Gain/1
  Delay3/1 -> Modulo by Constant HDL Optimized/1
  Delay4/1 -> Trigonometric Function/1
  Delay5/1 -> Product1/2

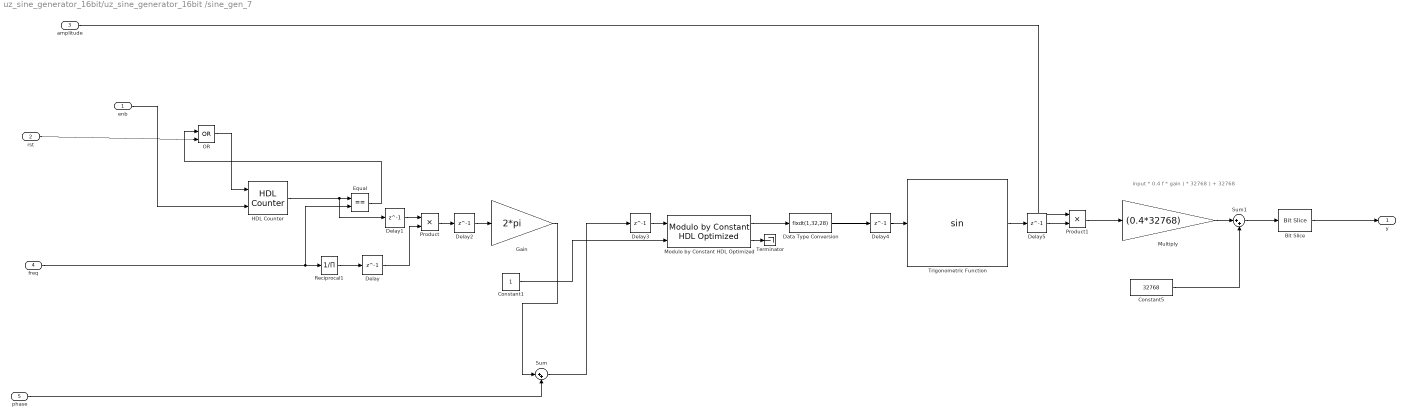
== system uz_sine_generator_16bit/uz_sine_generator_16bit /sine_gen_7 ==
  note: input * 0.4 f * gain ) * 32768 ) + 32768
  enb : Inport
  rst : Inport  Port=2
  amplitude : Inport  Port=3
  freq : Inport  Port=4
  phase : Inport  Port=5
  Bit Slice : hdlsllib/Logic and Bit Operations/Bit Slice  lidx=15  ridx=0
  Constant1 : Constant  OutDataTypeStr=boolean  SampleTime=-1
  Constant5 : Constant  Value=32768  OutDataTypeStr=int32  SampleTime=-1
  Data Type Conversion : DataTypeConversion  OutDataTypeStr=fixdt(1,32,28)  SaturateOnIntegerOverflow=off  RndMeth=Floor
  Delay{,1..5} (6 alike) : Delay  DelayLength=1
  Equal : RelationalOperator  Operator===  OutDataTypeStr=boolean  RndMeth=Simplest  InputSameDT=off
  Gain : Gain  Gain=2*pi  OutDataTypeStr=fixdt(1,32,28)
  HDL Counter : hdlsllib/Sources/HDL Counter  CountType=Free running  CountInit=0  CountStep=1  CountMax=25  CountFromType=Initial value  CountFrom=0  CountResetPort=on  CountLoadPort=off  CountEnbPort=on  CountDirPort=off  CountHitOutputPort=off  CountDataType=Unsigned  CountWordLen=32  CountFracLen=0  CountSampTime=1
  Modulo by Constant HDL Optimized : embmathops/Modulo by Constant HDL Optimized  Denominator=2*pi  SimulateUsing=Code generation
      settings: LibrarySourceBlock=|
      | embeddedMatrixLib/Math Operations/Modulo by Constant
      | HDL Optimized
  Multiply : Gain  Gain=(0.4*32768)  OutDataTypeStr=int32
  OR : Logic  Operator=OR  IconShape=distinctive  AllPortsSameDT=off  OutDataTypeStr=boolean
  Product : Product  OutDataTypeStr=fixdt(0,32,29)
  Product1 : Product  OutDataTypeStr=Inherit: Same as first input
  Reciprocal1 : Product  Inputs=/  RndMeth=Zero  SaturateOnIntegerOverflow=on
  Sum : Sum  Inputs=|++
  Sum1 : Sum  Inputs=|++  OutDataTypeStr=int32
  Terminator : Terminator
  Trigonometric Function : Trigonometry  ApproximationMethod=CORDIC
  y : Outport
  wires:
  Constant1/1 -> Modulo by Constant HDL Optimized/2
  Product1/1 -> Multiply/1
  Constant5/1 -> Sum1/2
  Gain/1 -> Sum/1
  Sum/1 -> Delay3/1
  Modulo by Constant HDL Optimized/1 -> Data Type Conversion/1
  freq/1 -> Reciprocal1/1, Equal/2
  Reciprocal1/1 -> Delay/1
  amplitude/1 -> Product1/1
  Sum1/1 -> Bit Slice/1
  phase/1 -> Sum/2
  Product/1 -> Delay2/1
  Equal/1 -> OR/1
  Trigonometric Function/1 -> Delay5/1
  enb/1 -> HDL Counter/2
  Multiply/1 -> Sum1/1
  Bit Slice/1 -> y/1
  Modulo by Constant HDL Optimized/2 -> Terminator/1
  OR/1 -> HDL Counter/1
  rst/1 -> OR/2
  HDL Counter/1 -> Delay1/1, Equal/1
  Data Type Conversion/1 -> Delay4/1
  Delay/1 -> Product/2
  Delay1/1 -> Product/1
  Delay2/1 -> Gain/1
  Delay3/1 -> Modulo by Constant HDL Optimized/1
  Delay4/1 -> Trigonometric Function/1
  Delay5/1 -> Product1/2

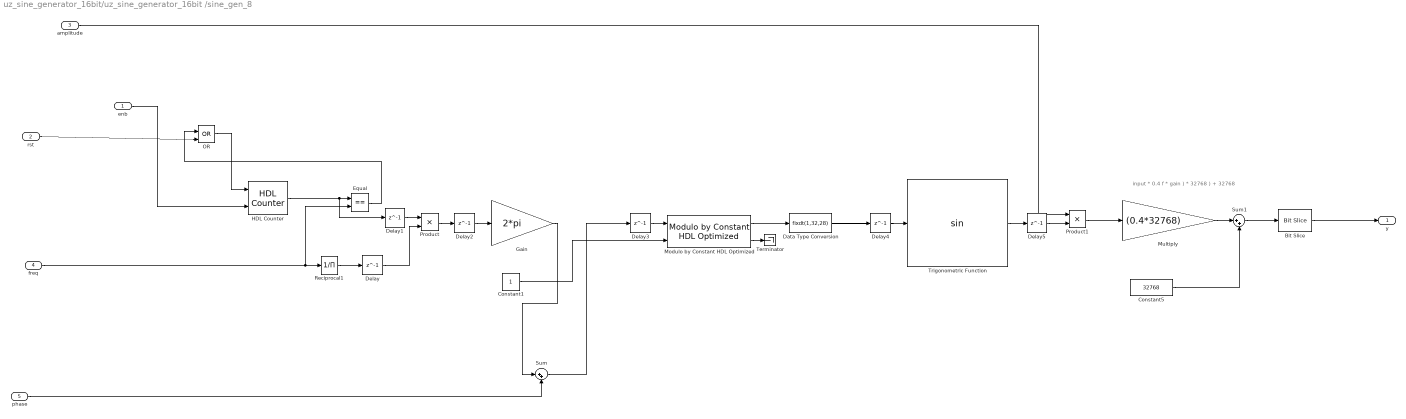
== system uz_sine_generator_16bit/uz_sine_generator_16bit /sine_gen_8 ==
  note: input * 0.4 f * gain ) * 32768 ) + 32768
  enb : Inport
  rst : Inport  Port=2
  amplitude : Inport  Port=3
  freq : Inport  Port=4
  phase : Inport  Port=5
  Bit Slice : hdlsllib/Logic and Bit Operations/Bit Slice  lidx=15  ridx=0
  Constant1 : Constant  OutDataTypeStr=boolean  SampleTime=-1
  Constant5 : Constant  Value=32768  OutDataTypeStr=int32  SampleTime=-1
  Data Type Conversion : DataTypeConversion  OutDataTypeStr=fixdt(1,32,28)  SaturateOnIntegerOverflow=off  RndMeth=Floor
  Delay{,1..5} (6 alike) : Delay  DelayLength=1
  Equal : RelationalOperator  Operator===  OutDataTypeStr=boolean  RndMeth=Simplest  InputSameDT=off
  Gain : Gain  Gain=2*pi  OutDataTypeStr=fixdt(1,32,28)
  HDL Counter : hdlsllib/Sources/HDL Counter  CountType=Free running  CountInit=0  CountStep=1  CountMax=25  CountFromType=Initial value  CountFrom=0  CountResetPort=on  CountLoadPort=off  CountEnbPort=on  CountDirPort=off  CountHitOutputPort=off  CountDataType=Unsigned  CountWordLen=32  CountFracLen=0  CountSampTime=1
  Modulo by Constant HDL Optimized : embmathops/Modulo by Constant HDL Optimized  Denominator=2*pi  SimulateUsing=Code generation
      settings: LibrarySourceBlock=|
      | embeddedMatrixLib/Math Operations/Modulo by Constant
      | HDL Optimized
  Multiply : Gain  Gain=(0.4*32768)  OutDataTypeStr=int32
  OR : Logic  Operator=OR  IconShape=distinctive  AllPortsSameDT=off  OutDataTypeStr=boolean
  Product : Product  OutDataTypeStr=fixdt(0,32,29)
  Product1 : Product  OutDataTypeStr=Inherit: Same as first input
  Reciprocal1 : Product  Inputs=/  RndMeth=Zero  SaturateOnIntegerOverflow=on
  Sum : Sum  Inputs=|++
  Sum1 : Sum  Inputs=|++  OutDataTypeStr=int32
  Terminator : Terminator
  Trigonometric Function : Trigonometry  ApproximationMethod=CORDIC
  y : Outport
  wires:
  Constant1/1 -> Modulo by Constant HDL Optimized/2
  Product1/1 -> Multiply/1
  Constant5/1 -> Sum1/2
  Gain/1 -> Sum/1
  Sum/1 -> Delay3/1
  Modulo by Constant HDL Optimized/1 -> Data Type Conversion/1
  freq/1 -> Reciprocal1/1, Equal/2
  Reciprocal1/1 -> Delay/1
  amplitude/1 -> Product1/1
  Sum1/1 -> Bit Slice/1
  phase/1 -> Sum/2
  Product/1 -> Delay2/1
  Equal/1 -> OR/1
  Trigonometric Function/1 -> Delay5/1
  enb/1 -> HDL Counter/2
  Multiply/1 -> Sum1/1
  Bit Slice/1 -> y/1
  Modulo by Constant HDL Optimized/2 -> Terminator/1
  OR/1 -> HDL Counter/1
  rst/1 -> OR/2
  HDL Counter/1 -> Delay1/1, Equal/1
  Data Type Conversion/1 -> Delay4/1
  Delay/1 -> Product/2
  Delay1/1 -> Product/1
  Delay2/1 -> Gain/1
  Delay3/1 -> Modulo by Constant HDL Optimized/1
  Delay4/1 -> Trigonometric Function/1
  Delay5/1 -> Product1/2
